simulink model "hexAeroTestHarness"  (R2024a)
settings: configuration reference "standardSILConfiguraitonParams" (kept outside this file)
settings Model: Creator=jerem  LastModifiedBy=jerem
settings ConfigSetRef: SourceName=standardSILConfiguraitonParams  SourceLocation=Base Workspace

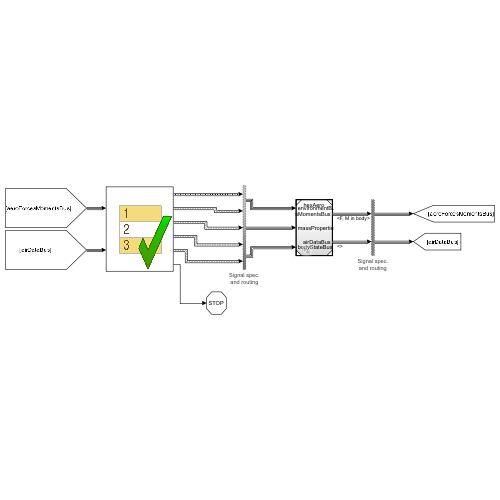
[thumbnail: Simulink's stored preview of the top-level diagram]
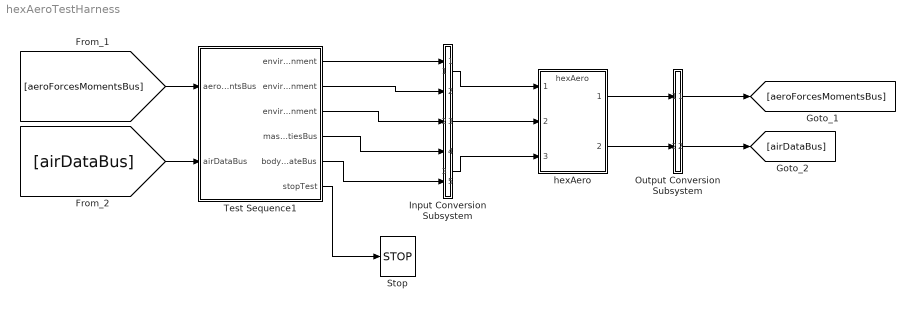
== system hexAeroTestHarness ==
  Input Conversion Subsystem : Subsystem  Tag=__SLT_ICS__  Description=|
      | Signal spec.
      | and routing
      settings: AttributesFormatString=%<Description>
  Output Conversion Subsystem : Subsystem  Tag=__SLT_OCS__  Description=|
      | Signal spec.
      | and routing
      mask init:
      | ICDictionary = get_param(bdroot, 'DataDictionary');
      | if isempty(ICDictionary)
      |    ICScope = Simulink.data.BaseWorkspace;
      | else
      |    ICScope = Simulink.data.DataDictionary(ICDictionary);
      | end
      | 
      | IC1 = Simulink.Bus.createMATLABStruct('ComponentForcesMomentsBus', [], [1 1], ICScope);
      | IC2 = Simulink.Bus.createMATLABStruct('AirDataBus', [], [1 1], ICScope);
      settings: AttributesFormatString=%<Description>
  Stop : Stop
  Test Sequence1 : Test Sequence  TreatAsAtomicUnit=on
  hexAero : ModelReference  ModelNameDialog=hexAero  SimulationMode=Normal  ModelReferenceVersion=1.15
  wires:
  Test Sequence1/1(environmentBus_EarthEnvironment) -> Input Conversion Subsystem/1(Inport_1)
  Test Sequence1/2(environmentBus_AirEnvironment) -> Input Conversion Subsystem/2(Inport_2)
  Test Sequence1/3(environmentBus_TerrainEnvironment) -> Input Conversion Subsystem/3(Inport_3)
  Test Sequence1/4(massPropertiesBus) -> Input Conversion Subsystem/4(Inport_4)
  Test Sequence1/5(bodyStateBus) -> Input Conversion Subsystem/5(Inport_5)
  [aeroForcesMomentsBus] -> Test Sequence1/1(aeroForcesMomentsBus)
  [airDataBus] -> Test Sequence1/2(airDataBus)
  Output Conversion Subsystem/1(Outport_1) -> [aeroForcesMomentsBus]
  Output Conversion Subsystem/2(Outport_2) -> [airDataBus]
  Input Conversion Subsystem/1(Outport_1) -> hexAero/1
  Input Conversion Subsystem/2(Outport_2) -> hexAero/2
  Input Conversion Subsystem/3(Outport_3) -> hexAero/3
  hexAero/1 -> Output Conversion Subsystem/1(Inport_1)
  hexAero/2 -> Output Conversion Subsystem/2(Inport_2)
  Test Sequence1/6(stopTest) -> Stop/1

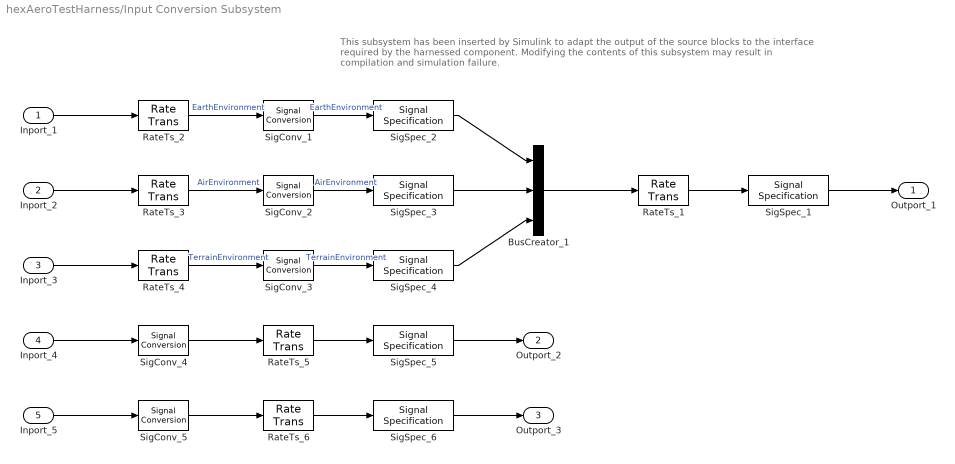
== system hexAeroTestHarness/Input Conversion Subsystem ==
  note: This subsystem has been inserted by Simulink to adapt the output of the source blocks to the interface required by the harnessed component.
      |  Modifying the contents of this subsystem may result in compilation and simulation failure.
  Inport_1 : Inport
  Inport_2 : Inport  Port=2
  Inport_3 : Inport  Port=3
  Inport_4 : Inport  Port=4
  Inport_5 : Inport  Port=5
  BusCreator_1 : BusCreator  Inputs=3  OutDataTypeStr=Bus: EnvironmentBus
  RateTs_{1..6} (6 alike) : RateTransition  OutPortSampleTime=0.004
  SigConv_1 : SignalConversion  ConversionOutput=Nonvirtual bus  OverrideOpt=off
  SigConv_2 : SignalConversion  ConversionOutput=Nonvirtual bus  OverrideOpt=off
  SigConv_3 : SignalConversion  ConversionOutput=Nonvirtual bus  OverrideOpt=off
  SigConv_4 : SignalConversion  ConversionOutput=Virtual bus  OverrideOpt=off
  SigConv_5 : SignalConversion  ConversionOutput=Virtual bus  OverrideOpt=off
  SigSpec_1 : SignalSpecification  OutDataTypeStr=Bus: EnvironmentBus  SampleTime=0.004
  SigSpec_2 : SignalSpecification  OutDataTypeStr=Bus: EarthEnvironmentBus  Dimensions=[1]  SampleTime=0.004  BusOutputAsStruct=on
  SigSpec_3 : SignalSpecification  OutDataTypeStr=Bus: AirEnvironmentBus  Dimensions=[1]  SampleTime=0.004  BusOutputAsStruct=on
  SigSpec_4 : SignalSpecification  OutDataTypeStr=Bus: TerrainEnvironmentBus  Dimensions=[1]  SampleTime=0.004  BusOutputAsStruct=on
  SigSpec_5 : SignalSpecification  OutDataTypeStr=Bus: MassPropertiesBus  SampleTime=0.004
  SigSpec_6 : SignalSpecification  OutDataTypeStr=Bus: BodyStateBus  SampleTime=0.004
  Outport_1 : Outport
  Outport_2 : Outport  Port=2
  Outport_3 : Outport  Port=3
  wires:
  SigSpec_1/1 -> Outport_1/1
  RateTs_1/1 -> SigSpec_1/1
  BusCreator_1/1 -> RateTs_1/1
  SigSpec_2/1 -> BusCreator_1/1
  SigConv_1/1 -> SigSpec_2/1  "EarthEnvironment"
  RateTs_2/1 -> SigConv_1/1  "EarthEnvironment"
  Inport_1/1 -> RateTs_2/1
  SigSpec_3/1 -> BusCreator_1/2
  SigConv_2/1 -> SigSpec_3/1  "AirEnvironment"
  RateTs_3/1 -> SigConv_2/1  "AirEnvironment"
  Inport_2/1 -> RateTs_3/1
  SigSpec_4/1 -> BusCreator_1/3
  SigConv_3/1 -> SigSpec_4/1  "TerrainEnvironment"
  RateTs_4/1 -> SigConv_3/1  "TerrainEnvironment"
  Inport_3/1 -> RateTs_4/1
  SigSpec_5/1 -> Outport_2/1
  RateTs_5/1 -> SigSpec_5/1
  SigConv_4/1 -> RateTs_5/1
  Inport_4/1 -> SigConv_4/1
  SigSpec_6/1 -> Outport_3/1
  RateTs_6/1 -> SigSpec_6/1
  SigConv_5/1 -> RateTs_6/1
  Inport_5/1 -> SigConv_5/1

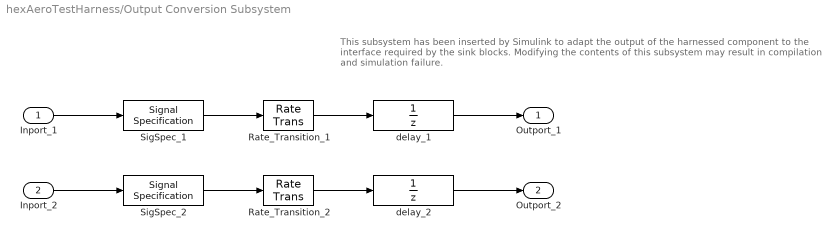
== system hexAeroTestHarness/Output Conversion Subsystem ==
  note: This subsystem has been inserted by Simulink to adapt the output of the harnessed component to the interface required by the sink blocks.
      |  Modifying the contents of this subsystem may result in compilation and simulation failure.
  Inport_1 : Inport
  Inport_2 : Inport  Port=2
  Rate_Transition_1 : RateTransition  OutPortSampleTimeOpt=Inherit
  Rate_Transition_2 : RateTransition  OutPortSampleTimeOpt=Inherit
  SigSpec_1 : SignalSpecification  OutDataTypeStr=Bus: ComponentForcesMomentsBus  Dimensions=[1]  SampleTime=0.004
  SigSpec_2 : SignalSpecification  OutDataTypeStr=Bus: AirDataBus  Dimensions=[1]  SampleTime=0.004
  delay_1 : UnitDelay  InitialCondition=IC1  SampleTime=-1
  delay_2 : UnitDelay  InitialCondition=IC2  SampleTime=-1
  Outport_1 : Outport
  Outport_2 : Outport  Port=2
  wires:
  Inport_1/1 -> SigSpec_1/1
  SigSpec_1/1 -> Rate_Transition_1/1
  Rate_Transition_1/1 -> delay_1/1
  delay_1/1 -> Outport_1/1
  Inport_2/1 -> SigSpec_2/1
  SigSpec_2/1 -> Rate_Transition_2/1
  Rate_Transition_2/1 -> delay_2/1
  delay_2/1 -> Outport_2/1

== stateflow chart hexAeroTestHarness/Test Sequence1 ==
  state Scenario_1
    state Initialize
      %% Initialize data outputs.
      environmentBus_EarthEnvironment.gravityScalar_mps2 = 0;
      environmentBus_EarthEnvironment.worldMagneticFieldInNED_nT = zeros(3,1);
      environmentBus_EarthEnvironment.mulh = zeros(3,1);
      environmentBus_AirEnvironment.airTemperature_K = 0;
      environmentBus_AirEnvironment.airPressure_Pa = 0;
      environmentBus_AirEnvironment.airDensity_kgpm3 = 0;
      environmentBus_AirEnvironment.windSpeedInNED_mps = zeros(3,1);
      environmentBus_AirEnvironment.speedOfSound_mps = 0;
      environmentBus_AirEnvironment.windsAloftInNED_mps = zeros(3,1);
      environmentBus_AirEnvironment.gustInNED_mps = zeros(3,1);
      environmentBus_AirEnvironment.turbulenceInNED_mps = zeros(3,1);
      environmentBus_TerrainEnvironment.terrainHeightInNED_m = 0;
      massPropertiesBus.aircraftMass_kg = 0;
      massPropertiesBus.aircraftCg_m = zeros(3,1);
      massPropertiesBus.aircraftInertiaInBody_kgm2 = zeros(3,3);
      massPropertiesBus.fuelLevelFraction = 0;
      bodyStateBus.aircraftVelInNED_mps = zeros(3,1);
      bodyStateBus.aircraftPosInNED_m = zeros(3,1);
      bodyStateBus.aircraftEulerAngles_rad = zeros(3,1);
      bodyStateBus.aircraftVelInBody_mps = zeros(3,1);
      bodyStateBus.aircraftAngVelInBody_radps = zeros(3,1);
      bodyStateBus.aircraftAngAccelInBody_radps2 = zeros(3,1);
      bodyStateBus.aircraftAccelInBody_mps2 = zeros(3,1);
      bodyStateBus.DCM_be = zeros(3,3);
      bodyStateBus.aircraftAccelbe_mps2 = zeros(3,1);
      stopTest = false;
    state SetDnPitchNoYaw
      environmentBus_AirEnvironment.airPressure_Pa = 101325;
      environmentBus_AirEnvironment.airDensity_kgpm3 = 1.225;
      bodyStateBus.aircraftVelInBody_mps = [10 0 -1]';
      yaw = 0;
      pitch = -0.1;
      eul = [yaw, pitch, 0]; % ZYX order, in radians
      bodyStateBus.DCM_be = eul2rotm(eul, 'ZYX')';
    state CheckDnPitchNoYaw
      %alpha_rad = -0.1
      %beta_rad = 0
      %FX -
      %FY 0
      %FZ +
      %MX 0
      %MY 0
      %MZ 0
      verify(aeroForcesMomentsBus.forcesInBody_N(1) < 0)
      verify(isClose(aeroForcesMomentsBus.forcesInBody_N(2), 0))
      verify(aeroForcesMomentsBus.forcesInBody_N(3) > 0)
      verify(isClose(aeroForcesMomentsBus.momentsInBody_Nm(1), 0))
      verify(isClose(aeroForcesMomentsBus.momentsInBody_Nm(2), 0))
      verify(isClose(aeroForcesMomentsBus.momentsInBody_Nm(3), 0))
      verify(isClose(airDataBus.airspeedInBody_mps(1), 10))
      verify(isClose(airDataBus.airspeedInBody_mps(2), 0))
      verify(isClose(airDataBus.airspeedInBody_mps(3), -1))
      verify(isClose(airDataBus.alpha_rad, -0.1, 'rtol',0.01))
      verify(isClose(airDataBus.beta_rad, 0, 'rtol',0.01))
    state SetUpPitchNoYaw
      bodyStateBus.aircraftVelInBody_mps = [10 0 1]';
      yaw = 0;
      pitch = 0.1;
      eul = [yaw, pitch, 0]; % ZYX order, in radians
      bodyStateBus.DCM_be = eul2rotm(eul, 'ZYX')';
    state CheckUpPitchNoYaw
      %alpha_rad = 0.1
      %beta_rad = 0
      %FX -
      %FY 0
      %FZ -
      %MX 0
      %MY 0
      %MZ 0
      verify(aeroForcesMomentsBus.forcesInBody_N(1) < 0)
      verify(isClose(aeroForcesMomentsBus.forcesInBody_N(2), 0))
      verify(aeroForcesMomentsBus.forcesInBody_N(3) < 0)
      verify(isClose(aeroForcesMomentsBus.momentsInBody_Nm(1), 0))
      verify(isClose(aeroForcesMomentsBus.momentsInBody_Nm(2), 0))
      verify(isClose(aeroForcesMomentsBus.momentsInBody_Nm(3), 0))
      verify(isClose(airDataBus.airspeedInBody_mps(1), 10))
      verify(isClose(airDataBus.airspeedInBody_mps(2), 0))
      verify(isClose(airDataBus.airspeedInBody_mps(3), 1))
      verify(isClose(airDataBus.alpha_rad, 0.1, 'rtol',0.01))
      verify(isClose(airDataBus.beta_rad, 0, 'rtol',0.01))
    state SetDnPitchNoseLeft
      bodyStateBus.aircraftVelInBody_mps = [10 1 -1]';
      yaw = -0.1;
      pitch = -0.1;
      eul = [yaw, pitch, 0]; % ZYX order, in radians
      bodyStateBus.DCM_be = eul2rotm(eul, 'ZYX')';
    state CheckDnPitchNoseLeft
      %alpha_rad = -0.1
      %beta_rad = 0.1
      %FX -
      %FY -
      %FZ +
      %MX 0
      %MY 0
      %MZ 0
      verify(aeroForcesMomentsBus.forcesInBody_N(1) < 0)
      verify(aeroForcesMomentsBus.forcesInBody_N(2) < 0)
      verify(aeroForcesMomentsBus.forcesInBody_N(3) > 0)
      verify(isClose(aeroForcesMomentsBus.momentsInBody_Nm(1), 0))
      verify(isClose(aeroForcesMomentsBus.momentsInBody_Nm(2), 0))
      verify(isClose(aeroForcesMomentsBus.momentsInBody_Nm(3), 0))
      verify(isClose(airDataBus.airspeedInBody_mps(1), 10))
      verify(isClose(airDataBus.airspeedInBody_mps(2), 1))
      verify(isClose(airDataBus.airspeedInBody_mps(3), -1))
      verify(isClose(airDataBus.alpha_rad, -0.1, 'rtol',0.01))
      verify(isClose(airDataBus.beta_rad, 0.1, 'rtol',0.01))
    state SetDnPitchNoseRight
      bodyStateBus.aircraftVelInBody_mps = [10 -1 -1]';
      yaw = 0.1;
      pitch = -0.1;
      eul = [yaw, pitch, 0]; % ZYX order, in radians
      bodyStateBus.DCM_be = eul2rotm(eul, 'ZYX')';
    state CheckDnPitchNoseRight
      %alpha_rad = -0.1
      %beta_rad = -0.1
      %FX -
      %FY +
      %FZ +
      %MX 0
      %MY 0
      %MZ 0
      verify(aeroForcesMomentsBus.forcesInBody_N(1) < 0)
      verify(aeroForcesMomentsBus.forcesInBody_N(2) > 0)
      verify(aeroForcesMomentsBus.forcesInBody_N(3) > 0)
      verify(isClose(aeroForcesMomentsBus.momentsInBody_Nm(1), 0))
      verify(isClose(aeroForcesMomentsBus.momentsInBody_Nm(2), 0))
      verify(isClose(aeroForcesMomentsBus.momentsInBody_Nm(3), 0))
      verify(isClose(airDataBus.airspeedInBody_mps(1), 10))
      verify(isClose(airDataBus.airspeedInBody_mps(2), -1))
      verify(isClose(airDataBus.airspeedInBody_mps(3), -1))
      verify(isClose(airDataBus.alpha_rad, -0.1, 'rtol',0.01))
      verify(isClose(airDataBus.beta_rad, -0.1, 'rtol',0.01))
    state setUpPitchNoseRightAndWind
      % repeat similar tests but add wind
      bodyStateBus.aircraftVelInBody_mps = [0 0 0]';
      yaw = 0.1;
      pitch = 0.1;
      eul = [yaw, pitch, 0]; % ZYX order, in radians
      bodyStateBus.DCM_be = eul2rotm(eul, 'ZYX')';
      environmentBus_AirEnvironment.windSpeedInNED_mps = -[10 0 0 ]';
    state CheckUpPitchNoseRightWind
      %alpha_rad = 0.1
      %beta_rad = -0.1
      %FX -
      %FY +
      %FZ -
      %MX 0
      %MY 0
      %MZ 0
      verify(aeroForcesMomentsBus.forcesInBody_N(1) < 0)
      verify(aeroForcesMomentsBus.forcesInBody_N(2) > 0)
      verify(aeroForcesMomentsBus.forcesInBody_N(3) < 0)
      verify(isClose(aeroForcesMomentsBus.momentsInBody_Nm(1), 0))
      verify(isClose(aeroForcesMomentsBus.momentsInBody_Nm(2), 0))
      verify(isClose(aeroForcesMomentsBus.momentsInBody_Nm(3), 0))
      verify(isClose(airDataBus.airspeedInBody_mps(1), 10, 'rtol',0.1))
      verify(isClose(airDataBus.airspeedInBody_mps(2), -1, 'rtol',0.1))
      verify(isClose(airDataBus.airspeedInBody_mps(3), 1, 'rtol',0.1))
      verify(isClose(airDataBus.alpha_rad, 0.1, 'rtol',0.1))
      verify(isClose(airDataBus.beta_rad, -0.1, 'rtol',0.1))
    state EndTest
      stopTest = true;
    (default) -> Initialize
    Initialize -> SetDnPitchNoYaw : [
        | true
        | ]
    SetDnPitchNoYaw -> CheckDnPitchNoYaw : [
        | after(1, sec)
        | ]
    CheckDnPitchNoYaw -> SetUpPitchNoYaw : [
        | true
        | ]
    SetUpPitchNoYaw -> CheckUpPitchNoYaw : [
        | after(1, sec)
        | ]
    CheckUpPitchNoYaw -> SetDnPitchNoseLeft : [
        | true
        | ]
    SetDnPitchNoseLeft -> CheckDnPitchNoseLeft : [
        | after(1, sec)
        | ]
    CheckDnPitchNoseLeft -> SetDnPitchNoseRight : [
        | true
        | ]
    SetDnPitchNoseRight -> CheckDnPitchNoseRight : [
        | after(1, sec)
        | ]
    CheckDnPitchNoseRight -> setUpPitchNoseRightAndWind : [
        | true
        | ]
    setUpPitchNoseRightAndWind -> CheckUpPitchNoseRightWind : [
        | after(1, sec)
        | ]
    CheckUpPitchNoseRightWind -> EndTest : [
        | true
        | ]
  (default) -> Scenario_1 : {assert(Active_Scenario_Index == 1,'The value of Scenario Parameter ''Active_Scenario_Index'' is not valid. Use the index of the scenario to specify it.')}
  data: aeroForcesMomentsBus input Bus: ComponentForcesMomentsBus size=[1]; airDataBus input Bus: AirDataBus size=[1]; environmentBus_EarthEnvironment output Bus: EarthEnvironmentBus size=[1]; environmentBus_AirEnvironment output Bus: AirEnvironmentBus size=[1]; environmentBus_TerrainEnvironment output Bus: TerrainEnvironmentBus size=[1]; massPropertiesBus output Bus: MassPropertiesBus size=[1]; bodyStateBus output Bus: BodyStateBus size=[1]; stopTest output; Active_Scenario_Index parameter =1; eul local; yaw local; pitch local
